simulink model "UnforcedTest"  (R2025b)
settings: Solver=FixedStepAuto  StartTime=0.0  StopTime=10  FixedStep=Ts  MaxStep=0.015  RelTol=1e-3
StopFcn:
  | stopHeli_allTasks
  | daqreset
model workspace: external: MAT-File (data not in the file)
undefined symbols (not defined in the file or in its folder): DAC_lim_l, DAC_lim_u, DiscIntNeverNeededParam, ElevAxisData, PitchAxisData, Ts
libraries: sldrtlib x1
settings Model: Creator=msciola  LastModifiedBy=leeta
settings SolverCC: AlgebraicLoopSolver=TrustRegion
settings DebuggingCC: UnconnectedInputMsg=warning  UnconnectedOutputMsg=warning  UnconnectedLineMsg=warning
settings ModelReferenceCC: EnableRefExpFcnMdlSchedulingChecks=on
settings SFSimCC: CustomCodeUndefinedFunction=UseInterfaceOnly
settings RTWCC: GPUComputeCapability=3.5

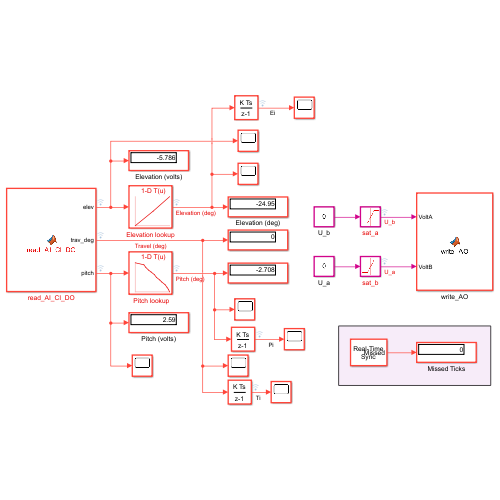
[thumbnail: Simulink's stored preview of the top-level diagram]
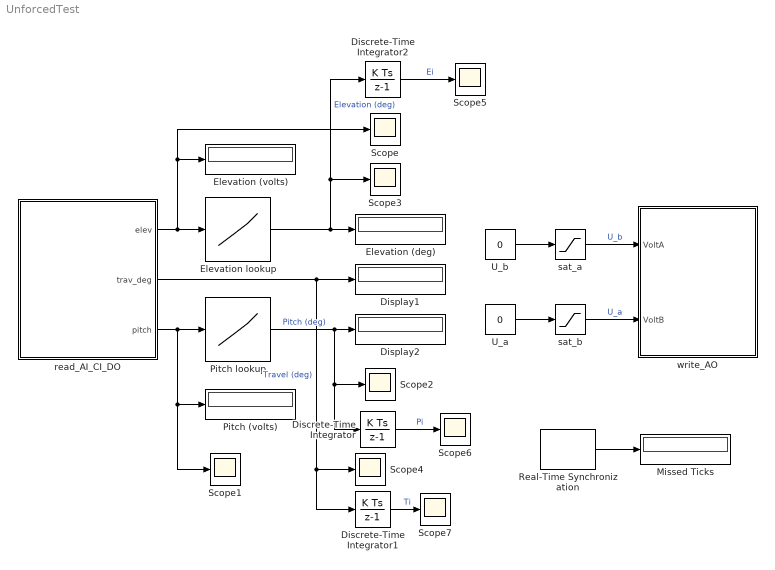
== system UnforcedTest ==
  " Pitch lookup" : Lookup_n-D  NumberOfTableDimensions=1  LookupTableObject=PitchAxisData  BreakpointsForDimension1=PitchAxisData.Var2  Table=PitchAxisData.Var1  InternalRulePriority=Speed  RndMeth=Simplest
  Discrete-Time Integrator : DiscreteIntegrator  SampleTime=Ts  ICPrevOutput=DiscIntNeverNeededParam  ICPrevScaledInput=DiscIntNeverNeededParam
  Discrete-Time Integrator1 : DiscreteIntegrator  SampleTime=Ts  ICPrevOutput=DiscIntNeverNeededParam  ICPrevScaledInput=DiscIntNeverNeededParam
  Discrete-Time Integrator2 : DiscreteIntegrator  SampleTime=Ts  ICPrevOutput=DiscIntNeverNeededParam  ICPrevScaledInput=DiscIntNeverNeededParam
  Display1 : Display
  Display2 : Display
  Elevation (deg) : Display
  Elevation (volts) : Display
  Elevation lookup : Lookup_n-D  NumberOfTableDimensions=1  LookupTableObject=PitchAxisData  BreakpointsForDimension1=ElevAxisData.Var2  Table=ElevAxisData.Var1  InternalRulePriority=Speed  RndMeth=Simplest
  Missed Ticks : Display
  Pitch (volts) : Display
  Real-Time Synchronization : sldrtlib/Real-Time Synchronization  SampleTime=Ts  MaxMissedTicks=inf  ShowMissedTicks=on  YieldWhenWaiting=off
  Scope{,1..7} (8 alike) : Scope
      Scope settings: ActiveDisplayYMinimum=1.9868510849967642  ActiveDisplayYMaximum=2.1934940167933932
      Scope1 settings: ActiveDisplayYMinimum=0.89176071528553269  ActiveDisplayYMaximum=2.568402255752348
      Scope2 settings: ActiveDisplayYMinimum=-12.003455637488393  ActiveDisplayYMaximum=16.21355916098214  DataLoggingVariableName=ScopeData2
      Scope3 settings: ActiveDisplayYMinimum=-26.137860483196686  ActiveDisplayYMaximum=-24.318243691799278  DataLoggingVariableName=ScopeData3
      Scope4 settings: ActiveDisplayYMinimum=-3.5457416169231357  ActiveDisplayYMaximum=4.3689375234098868  DataLoggingVariableName=ScopeData4
      Scope5 settings: ActiveDisplayYMinimum=-408.352580205493  ActiveDisplayYMaximum=101.7705588435243  DataLoggingVariableName=ScopeData5
      Scope6 settings: DataLoggingVariableName=ScopeData6
      Scope7 settings: DataLoggingVariableName=ScopeData7
  U_a : Constant  Value=0
  U_b : Constant  Value=0
  read_AI_CI_DO : MATLAB Function  TreatAsAtomicUnit=on
  sat_a : Saturate  UpperLimit=DAC_lim_u  LowerLimit=DAC_lim_l
  sat_b : Saturate  UpperLimit=DAC_lim_u  LowerLimit=DAC_lim_l
  write_AO : MATLAB Function  TreatAsAtomicUnit=on
  wires:
  Real-Time Synchronization/1 -> Missed Ticks/1
  read_AI_CI_DO/3(pitch) -> Scope1/1, Pitch (volts)/1, " Pitch lookup"/1
  read_AI_CI_DO/1(elev) -> Scope/1, Elevation (volts)/1, Elevation lookup/1
  read_AI_CI_DO/2(trav_deg) -> Discrete-Time Integrator1/1, Scope4/1, Display1/1  "Travel (deg)"
  Elevation lookup/1 -> Discrete-Time Integrator2/1, Scope3/1, Elevation (deg)/1  "Elevation (deg)"
  " Pitch lookup"/1 -> Discrete-Time Integrator/1, Scope2/1, Display2/1  "Pitch (deg)"
  U_b/1 -> sat_a/1
  sat_a/1 -> write_AO/1(VoltA)  "U_b"
  U_a/1 -> sat_b/1
  sat_b/1 -> write_AO/2(VoltB)  "U_a"
  Discrete-Time Integrator1/1 -> Scope7/1  "Ti"
  Discrete-Time Integrator/1 -> Scope6/1  "Pi"
  Discrete-Time Integrator2/1 -> Scope5/1  "Ei"

== matlab function UnforcedTest/read_AI_CI_DO ==
  data: elev output; trav_deg output; pitch output
function [elev,trav_deg,pitch] = read_AI_CI_DO()
% The functions from the NI library to read and write inputs and outpus 
% cannot be compiled and we need to use the coder.extrinsic.
% Functions in common to all 
coder.extrinsic('NI_DAQmxCreateTask','NI_DAQmxStartTask','assignin');
%Functions to read AI
coder.extrinsic('daq.ni.NIDAQmx.DAQmx_Val_Diff','NI_DAQmxCreateAIVoltageChan',...
    'NI_DAQmxReadAnalogF64');
%Functions to read CI
coder.extrinsic('NI_DAQmxCreateCILinEncoderChan','NI_DAQmxReadCounterScalarF64',... 
    'daq.ni.NIDAQmx.DAQmx_Val_X1','daq.ni.NIDAQmx.DAQmx_Val_Ticks');
%Functions to write DO
coder.extrinsic('NI_DAQmxWriteDigitalLines','NI_DAQmxCreateDOChan');

%% Configuration
% Specify channels
channelNameAI = {'myDAQ1/ai0','myDAQ1/ai1'};
channelNameCI = 'myDAQ1/ctr0';
channelNamesDO = {'myDAQ1/Port0/Line5', 'myDAQ1/Port0/Line6','myDAQ1/Port0/Line7'};

% Initialize variables for MATLAB Function block to work
elev = 0;
pitch = 0;
numChannels = 1;
trav = zeros(1, numChannels);
y = zeros(1, numChannels);
% make the taskhandle for each channel persistent
persistent taskHandleAI taskHandleCI taskHandleDO
% Create and start tasks for each channel
if isempty(taskHandleAI)
    taskHandleAI = NI_DAQmxCreateTask;
    NI_DAQmxCreateAIVoltageChan(taskHandleAI, channelNameAI{1}, daq.ni.NIDAQmx.DAQmx_Val_Diff, -10, 10)
    NI_DAQmxCreateAIVoltageChan(taskHandleAI, channelNameAI{2}, daq.ni.NIDAQmx.DAQmx_Val_Diff, -10, 10)
    NI_DAQmxStartTask(taskHandleAI);
    assignin('base','taskHandleAI',taskHandleAI);
end
if isempty(taskHandleCI)
    taskHandleCI = NI_DAQmxCreateTask;
    NI_DAQmxCreateCILinEncoderChan( taskHandleCI, channelNameCI, daq.ni.NIDAQmx.DAQmx_Val_X1, daq.ni.NIDAQmx.DAQmx_Val_Ticks, 1); % Check X4 (Labview) or X1 with Bryn
    NI_DAQmxStartTask(taskHandleCI)
    assignin('base','taskHandleCI',taskHandleCI);
end
if isempty (taskHandleDO)
    taskHandleDO = NI_DAQmxCreateTask;
    for ii = 1:numel(channelNamesDO)
        NI_DAQmxCreateDOChan(taskHandleDO, channelNamesDO{ii});
    end
    %numChannelsDO = NI_DAQmxGetWriteNumChans(taskHandleDO);
    NI_DAQmxStartTask(taskHandleDO)
    assignin('base','taskHandleDO',taskHandleDO);
end
%% Read and write channels
% Write the digital outputs
outputData = [0 1 0];
NI_DAQmxWriteDigitalLines(taskHandleDO, outputData);
% Read analog inputs (elevation and pitch angles)
data = NI_DAQmxReadAnalogF64(taskHandleAI,1,2);
elev = data(1);
pitch = data(2);

% Read the counter encoder input (tavel angle)
y = NI_DAQmxReadCounterScalarF64(taskHandleCI);
% To avoid insignificant numbers in the reading
if y> 2^31
    y = y- 2^32;
end
% Transform the encoder reading into angle degrees between 0 and 360
 trav_deg = y*360/500;
end

== matlab function UnforcedTest/write_AO ==
  data: VoltA input; VoltB input
function write_AO(VoltA,VoltB)
% The functions from the NI library to write outpus cannot be compiled 
% and we need to use the coder.extrinsic.
% Functions in common to all  
coder.extrinsic('NI_DAQmxCreateTask','NI_DAQmxStartTask', 'assignin');
% Functions to write AO
coder.extrinsic('NI_DAQmxCreateAOVoltageChan','NI_DAQmxWriteAnalogF64',...
    'daq.ni.NIDAQmx.DAQmx_Val_Volts');
%% Configuration
% Specify channel
channelNameAO = {'myDAQ1/ao0','myDAQ1/ao1'};
% make the taskhandle persistent
persistent  taskHandleAO 
% Create and start tasks for each channel
if isempty(taskHandleAO)
    taskHandleAO = NI_DAQmxCreateTask;
    NI_DAQmxCreateAOVoltageChan(taskHandleAO, channelNameAO{1})
    NI_DAQmxCreateAOVoltageChan(taskHandleAO, channelNameAO{2})
    NI_DAQmxStartTask(taskHandleAO);
    assignin('base','taskHandleAO',taskHandleAO);
end
%% Write Digital output
NI_DAQmxWriteAnalogF64(taskHandleAO,[VoltA,VoltB]);
end
